simulink model "g_s_cl3"  (Simulink 5.0)
settings: Solver=ode45  StartTime=t_init  StopTime=t_final  RelTol=1e-3
undefined symbols (not defined in the file or in its folder): den, den1, denb, denf, num, num1, numb, numf, st, st1, Ts
settings Model: Creator=kannan  LastModifiedBy=kannan  ExtModeAutoUpdateStatusClock=off

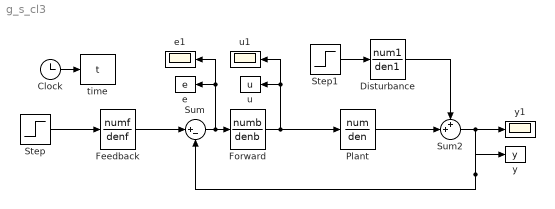
== system g_s_cl3 ==
  Clock : Clock
      settings: Decimation=10
  Disturbance : TransferFcn  Numerator=num1  Denominator=den1
  Feedback : TransferFcn  Numerator=numf  Denominator=denf
  Forward : TransferFcn  Numerator=numb  Denominator=denb
  Plant : TransferFcn  Numerator=num  Denominator=den
  Step : Step  Time=0  After=st  SampleTime=Ts
  Step1 : Step  Time=0  After=st1  SampleTime=Ts
  Sum : Sum  Inputs=|+-  SaturateOnIntegerOverflow=on
  Sum2 : Sum  Inputs=++|  SaturateOnIntegerOverflow=on
  e : ToWorkspace  VariableName=e  SampleTime=Ts  SaveFormat=Array
  e1 : Scope
      settings: YMin=-6e+164  YMax=1.02293e+149  SaveName=ScopeData2
  time : ToWorkspace  VariableName=t  SampleTime=Ts  SaveFormat=Array
  u : ToWorkspace  VariableName=u  SampleTime=Ts  SaveFormat=Array
  u1 : Scope
      settings: YMin=-6e+164  YMax=1.02293e+149
  y : ToWorkspace  VariableName=y  SampleTime=Ts  SaveFormat=Array
  y1 : Scope
      settings: YMin=-6e+164  YMax=1.02293e+149
  wires:
  Feedback/1 -> Sum/1
  Clock/1 -> time/1
  Plant/1 -> Sum2/2
  Disturbance/1 -> Sum2/1
  Step1/1 -> Disturbance/1
  Sum2/1 -> y1/1, y/1, Sum/2
  Sum/1 -> e/1, e1/1, Forward/1
  Forward/1 -> u1/1, u/1, Plant/1
  Step/1 -> Feedback/1
